simulink model "sm_i2c_expansion"  (Simulink 9.2)
settings: Solver=VariableStepAuto  StartTime=0.0  StopTime=10.0  RelTol=1e-3
undefined symbols (not defined in the file): slave_i2c
libraries: haley_test_bench_lib x10, etherlab_lib x1
settings Model: Creator=entwicklungs-pc  LastModifiedBy=entwicklungs-pc
settings DataIOCC: LimitDataPoints=off  SaveFormat=Dataset  SignalLoggingSaveFormat=Dataset
settings OptimizationCC: LifeSpan=auto
settings DebuggingCC: UnderspecifiedInitializationDetection=Simplified  MergeDetectMultiDrivingBlocksExec=error  FcnCallInpInsideContextMsg=error  StateNameClashWarn=none  SFUnexpectedBacktrackingDiag=error  SFNoUnconditionalDefaultTransitionDiag=error  SFExecutionAtInitializationDiag=warning
settings HardwareCC: ProdBitPerPointer=64  ProdBitPerSizeT=64  ProdBitPerPtrDiffT=64  ProdLargestAtomicFloat=Float  ProdIntDivRoundTo=Zero  ProdEndianess=LittleEndian  ProdWordSize=64  ProdHWDeviceType=Intel->x86-64 (Windows64)
settings ModelReferenceCC: PropagateSignalLabelsOutOfModel=on
settings SFSimCC: SimUseLocalCustomCode=on
settings RTWCC: RTWUseLocalCustomCode=on
settings CodeAppCC: StateflowObjectComments=off
settings GRTTargetCC: TargetLangStandard=C99 (ISO)  GeneratePreprocessorConditionals=Use local settings  CombineOutputUpdateFcns=on  GRTInterface=off
settings ConfigComp: CovMetricSettings=dwe  CovHtmlReporting=off  CovSaveCumulativeToWorkspaceVar=off  CovSaveSingleToWorkspaceVar=off  CovExternalEMLEnable=on

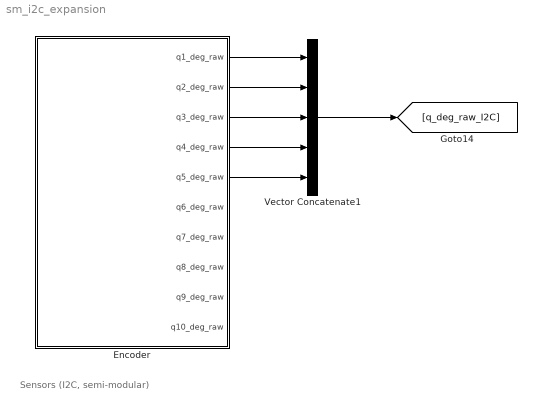
== system sm_i2c_expansion ==
  note: Sensors (I2C, semi-modular)
  Encoder : Subsystem
  Vector Concatenate1 : Concatenate  NumInputs=5
  wires:
  Encoder/1(q1_deg_raw) -> Vector Concatenate1/1
  Encoder/2(q2_deg_raw) -> Vector Concatenate1/2
  Encoder/5(q5_deg_raw) -> Vector Concatenate1/5
  Vector Concatenate1/1 -> [q_deg_raw_I2C]
  Encoder/3(q3_deg_raw) -> Vector Concatenate1/3
  Encoder/4(q4_deg_raw) -> Vector Concatenate1/4

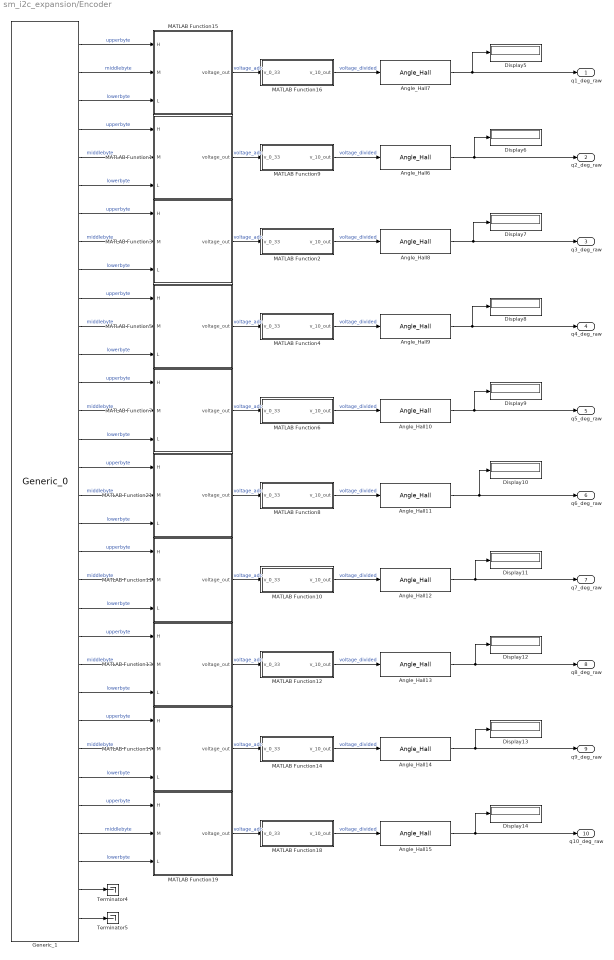
== system sm_i2c_expansion/Encoder ==
  Angle_Hall{6..15} (10 alike) : haley_test_bench_lib/Angle_Hall  SystemSampleTime=-1
  Display{5..14} (10 alike) : Display
  Generic_1 : etherlab_lib/EtherCAT/Generic_0  master=0  index=16  rv=slave_i2c()  param=[]  tsample=t_sample_s  debug=0
  MATLAB Function1 : MATLAB Function  TreatAsAtomicUnit=on
  MATLAB Function10 : MATLAB Function  TreatAsAtomicUnit=on
  MATLAB Function11 : MATLAB Function  TreatAsAtomicUnit=on
  MATLAB Function12 : MATLAB Function  TreatAsAtomicUnit=on
  MATLAB Function13 : MATLAB Function  TreatAsAtomicUnit=on
  MATLAB Function14 : MATLAB Function  TreatAsAtomicUnit=on
  MATLAB Function15 : MATLAB Function  TreatAsAtomicUnit=on
  MATLAB Function16 : MATLAB Function  TreatAsAtomicUnit=on
  MATLAB Function17 : MATLAB Function  TreatAsAtomicUnit=on
  MATLAB Function18 : MATLAB Function  TreatAsAtomicUnit=on
  MATLAB Function19 : MATLAB Function  TreatAsAtomicUnit=on
  MATLAB Function2 : MATLAB Function  TreatAsAtomicUnit=on
  MATLAB Function21 : MATLAB Function  TreatAsAtomicUnit=on
  MATLAB Function3 : MATLAB Function  TreatAsAtomicUnit=on
  MATLAB Function4 : MATLAB Function  TreatAsAtomicUnit=on
  MATLAB Function5 : MATLAB Function  TreatAsAtomicUnit=on
  MATLAB Function6 : MATLAB Function  TreatAsAtomicUnit=on
  MATLAB Function7 : MATLAB Function  TreatAsAtomicUnit=on
  MATLAB Function8 : MATLAB Function  TreatAsAtomicUnit=on
  MATLAB Function9 : MATLAB Function  TreatAsAtomicUnit=on
  Terminator4 : Terminator
  Terminator5 : Terminator
  q1_deg_raw : Outport
  q2_deg_raw : Outport  Port=2
  q3_deg_raw : Outport  Port=3
  q4_deg_raw : Outport  Port=4
  q5_deg_raw : Outport  Port=5
  q6_deg_raw : Outport  Port=6
  q7_deg_raw : Outport  Port=7
  q8_deg_raw : Outport  Port=8
  q9_deg_raw : Outport  Port=9
  q10_deg_raw : Outport  Port=10
  wires:
  MATLAB Function6/1(v_10_out) -> Angle_Hall10/1  "voltage_divided"
  Generic_1/3 -> MATLAB Function15/3(L)  "lowerbyte"
  Angle_Hall10/1 -> Display9/1, q5_deg_raw/1
  Angle_Hall6/1 -> q2_deg_raw/1, Display6/1
  MATLAB Function3/1(voltage_out) -> MATLAB Function2/1(v_0_33)  "voltage_adc"
  MATLAB Function2/1(v_10_out) -> Angle_Hall8/1  "voltage_divided"
  Generic_1/4 -> MATLAB Function1/1(H)  "upperbyte"
  Angle_Hall8/1 -> q3_deg_raw/1, Display7/1
  Generic_1/6 -> MATLAB Function1/3(L)  "lowerbyte"
  Generic_1/1 -> MATLAB Function15/1(H)  "upperbyte"
  MATLAB Function15/1(voltage_out) -> MATLAB Function16/1(v_0_33)  "voltage_adc"
  Generic_1/2 -> MATLAB Function15/2(M)  "middlebyte"
  Angle_Hall7/1 -> q1_deg_raw/1, Display5/1
  Generic_1/9 -> MATLAB Function3/3(L)  "lowerbyte"
  MATLAB Function5/1(voltage_out) -> MATLAB Function4/1(v_0_33)  "voltage_adc"
  MATLAB Function7/1(voltage_out) -> MATLAB Function6/1(v_0_33)  "voltage_adc"
  Generic_1/8 -> MATLAB Function3/2(M)  "middlebyte"
  MATLAB Function4/1(v_10_out) -> Angle_Hall9/1  "voltage_divided"
  MATLAB Function16/1(v_10_out) -> Angle_Hall7/1  "voltage_divided"
  MATLAB Function1/1(voltage_out) -> MATLAB Function9/1(v_0_33)  "voltage_adc"
  Generic_1/7 -> MATLAB Function3/1(H)  "upperbyte"
  Generic_1/10 -> MATLAB Function5/1(H)  "upperbyte"
  Generic_1/12 -> MATLAB Function5/3(L)  "lowerbyte"
  Angle_Hall9/1 -> q4_deg_raw/1, Display8/1
  Generic_1/13 -> MATLAB Function7/1(H)  "upperbyte"
  Generic_1/15 -> MATLAB Function7/3(L)  "lowerbyte"
  MATLAB Function9/1(v_10_out) -> Angle_Hall6/1  "voltage_divided"
  Generic_1/11 -> MATLAB Function5/2(M)  "middlebyte"
  Generic_1/14 -> MATLAB Function7/2(M)  "middlebyte"
  Generic_1/5 -> MATLAB Function1/2(M)  "middlebyte"
  Generic_1/16 -> MATLAB Function21/1(H)  "upperbyte"
  Generic_1/28 -> MATLAB Function19/1(H)  "upperbyte"
  MATLAB Function11/1(voltage_out) -> MATLAB Function10/1(v_0_33)  "voltage_adc"
  Generic_1/27 -> MATLAB Function17/3(L)  "lowerbyte"
  Generic_1/22 -> MATLAB Function13/1(H)  "upperbyte"
  MATLAB Function13/1(voltage_out) -> MATLAB Function12/1(v_0_33)  "voltage_adc"
  Generic_1/23 -> MATLAB Function13/2(M)  "middlebyte"
  Generic_1/20 -> MATLAB Function11/2(M)  "middlebyte"
  Generic_1/18 -> MATLAB Function21/3(L)  "lowerbyte"
  MATLAB Function19/1(voltage_out) -> MATLAB Function18/1(v_0_33)  "voltage_adc"
  Generic_1/29 -> MATLAB Function19/2(M)  "middlebyte"
  Generic_1/26 -> MATLAB Function17/2(M)  "middlebyte"
  Generic_1/21 -> MATLAB Function11/3(L)  "lowerbyte"
  MATLAB Function17/1(voltage_out) -> MATLAB Function14/1(v_0_33)  "voltage_adc"
  Generic_1/19 -> MATLAB Function11/1(H)  "upperbyte"
  MATLAB Function14/1(v_10_out) -> Angle_Hall14/1  "voltage_divided"
  Angle_Hall11/1 -> q6_deg_raw/1, Display10/1
  MATLAB Function21/1(voltage_out) -> MATLAB Function8/1(v_0_33)  "voltage_adc"
  Angle_Hall15/1 -> q10_deg_raw/1, Display14/1
  Generic_1/24 -> MATLAB Function13/3(L)  "lowerbyte"
  MATLAB Function18/1(v_10_out) -> Angle_Hall15/1  "voltage_divided"
  Generic_1/30 -> MATLAB Function19/3(L)  "lowerbyte"
  Generic_1/17 -> MATLAB Function21/2(M)  "middlebyte"
  MATLAB Function12/1(v_10_out) -> Angle_Hall13/1  "voltage_divided"
  Generic_1/25 -> MATLAB Function17/1(H)  "upperbyte"
  Angle_Hall12/1 -> q7_deg_raw/1, Display11/1
  MATLAB Function8/1(v_10_out) -> Angle_Hall11/1  "voltage_divided"
  Angle_Hall13/1 -> q8_deg_raw/1, Display12/1
  Angle_Hall14/1 -> q9_deg_raw/1, Display13/1
  MATLAB Function10/1(v_10_out) -> Angle_Hall12/1  "voltage_divided"
  Generic_1/32 -> Terminator5/1
  Generic_1/31 -> Terminator4/1

== matlab function Encoder/MATLAB Function1 ==
  data: H input uint8 size=1; M input double; L input uint8 size=1; voltage_out output double size=1
function voltage_out = concat_bitwise(H, M, L)

    raw_value = double(bitshift(int32(H), 16) + bitshift(int32(M), 8) + int32(L));  

    % Convert raw ADC value to voltage
    voltage_out = (3.333333333333333333 / 8388607) * raw_value; 
end

== matlab function Encoder/MATLAB Function2 ==
  data: v_0_33 input double; v_10_out output double
function v_10_out = map_voltage(v_0_33)
%reconstruct output voltage after voltage divider
v_10_out = v_0_33*(1+2)/1; %divider: V_0_33 = V_10*R_2/(R_1+R_2) --- R1 = 200kOhm, R2=100kOhm

== matlab function Encoder/MATLAB Function3 ==
  data: H input uint8 size=1; M input double; L input uint8 size=1; voltage_out output double size=1
function voltage_out = concat_bitwise(H, M, L)

    raw_value = double(bitshift(int32(H), 16) + bitshift(int32(M), 8) + int32(L));  

    % Convert raw ADC value to voltage
    voltage_out = (3.333333333333333333 / 8388607) * raw_value; 
end

== matlab function Encoder/MATLAB Function4 ==
  data: v_0_33 input double; v_10_out output double
function v_10_out = map_voltage(v_0_33)
%reconstruct output voltage after voltage divider
v_10_out = v_0_33*(1+2)/1; %divider: V_0_33 = V_10*R_2/(R_1+R_2) --- R1 = 200kOhm, R2=100kOhm

== matlab function Encoder/MATLAB Function5 ==
  data: H input uint8 size=1; M input double; L input uint8 size=1; voltage_out output double size=1
function voltage_out = concat_bitwise(H, M, L)

    raw_value = double(bitshift(int32(H), 16) + bitshift(int32(M), 8) + int32(L));  

    % Convert raw ADC value to voltage
    voltage_out = (3.333333333333333333 / 8388607) * raw_value; 
end

== matlab function Encoder/MATLAB Function6 ==
  data: v_0_33 input double; v_10_out output double
function v_10_out = map_voltage(v_0_33)
%reconstruct output voltage after voltage divider
v_10_out = v_0_33*(1+2)/1; %divider: V_0_33 = V_10*R_2/(R_1+R_2) --- R1 = 200kOhm, R2=100kOhm

== matlab function Encoder/MATLAB Function7 ==
  data: H input uint8 size=1; M input double; L input uint8 size=1; voltage_out output double size=1
function voltage_out = concat_bitwise(H, M, L)

    raw_value = double(bitshift(int32(H), 16) + bitshift(int32(M), 8) + int32(L));  

    % Convert raw ADC value to voltage
    voltage_out = (3.333333333333333333 / 8388607) * raw_value; 
end

== matlab function Encoder/MATLAB Function8 ==
  data: v_0_33 input double; v_10_out output double
function v_10_out = map_voltage(v_0_33)
%reconstruct output voltage after voltage divider
v_10_out = v_0_33*(1+2)/1; %divider: V_0_33 = V_10*R_2/(R_1+R_2) --- R1 = 200kOhm, R2=100kOhm

== matlab function Encoder/MATLAB Function9 ==
  data: v_0_33 input double; v_10_out output double
function v_10_out = map_voltage(v_0_33)
%reconstruct output voltage after voltage divider
v_10_out = v_0_33*(1+2)/1; %divider: V_0_33 = V_10*R_2/(R_1+R_2) --- R1 = 200kOhm, R2=100kOhm

== matlab function Encoder/MATLAB Function10 ==
  data: v_0_33 input double; v_10_out output double
function v_10_out = map_voltage(v_0_33)
%reconstruct output voltage after voltage divider
v_10_out = v_0_33*(1+2)/1; %divider: V_0_33 = V_10*R_2/(R_1+R_2) --- R1 = 200kOhm, R2=100kOhm

== matlab function Encoder/MATLAB Function11 ==
  data: H input uint8 size=1; M input double; L input uint8 size=1; voltage_out output double size=1
function voltage_out = concat_bitwise(H, M, L)

    raw_value = double(bitshift(int32(H), 16) + bitshift(int32(M), 8) + int32(L));  

    % Convert raw ADC value to voltage
    voltage_out = (3.333333333333333333 / 8388607) * raw_value; 
end

== matlab function Encoder/MATLAB Function21 ==
  data: H input uint8 size=1; M input double; L input uint8 size=1; voltage_out output double size=1
function voltage_out = concat_bitwise(H, M, L)

    raw_value = double(bitshift(int32(H), 16) + bitshift(int32(M), 8) + int32(L));  

    % Convert raw ADC value to voltage
    voltage_out = (3.333333333333333333 / 8388607) * raw_value; 
end

== matlab function Encoder/MATLAB Function12 ==
  data: v_0_33 input double; v_10_out output double
function v_10_out = map_voltage(v_0_33)
%reconstruct output voltage after voltage divider
v_10_out = v_0_33*(1+2)/1; %divider: V_0_33 = V_10*R_2/(R_1+R_2) --- R1 = 200kOhm, R2=100kOhm

== matlab function Encoder/MATLAB Function13 ==
  data: H input uint8 size=1; M input double; L input uint8 size=1; voltage_out output double size=1
function voltage_out = concat_bitwise(H, M, L)

    raw_value = double(bitshift(int32(H), 16) + bitshift(int32(M), 8) + int32(L));  

    % Convert raw ADC value to voltage
    voltage_out = (3.333333333333333333 / 8388607) * raw_value; 
end

== matlab function Encoder/MATLAB Function14 ==
  data: v_0_33 input double; v_10_out output double
function v_10_out = map_voltage(v_0_33)
%reconstruct output voltage after voltage divider
v_10_out = v_0_33*(1+2)/1; %divider: V_0_33 = V_10*R_2/(R_1+R_2) --- R1 = 200kOhm, R2=100kOhm

== matlab function Encoder/MATLAB Function17 ==
  data: H input uint8 size=1; M input double; L input uint8 size=1; voltage_out output double size=1
function voltage_out = concat_bitwise(H, M, L)

    raw_value = double(bitshift(int32(H), 16) + bitshift(int32(M), 8) + int32(L));  

    % Convert raw ADC value to voltage
    voltage_out = (3.333333333333333333 / 8388607) * raw_value; 
end

== matlab function Encoder/MATLAB Function18 ==
  data: v_0_33 input double; v_10_out output double
function v_10_out = map_voltage(v_0_33)
%reconstruct output voltage after voltage divider
v_10_out = v_0_33*(1+2)/1; %divider: V_0_33 = V_10*R_2/(R_1+R_2) --- R1 = 200kOhm, R2=100kOhm

== matlab function Encoder/MATLAB Function19 ==
  data: H input uint8 size=1; M input double; L input uint8 size=1; voltage_out output double size=1
function voltage_out = concat_bitwise(H, M, L)

    raw_value = double(bitshift(int32(H), 16) + bitshift(int32(M), 8) + int32(L));  

    % Convert raw ADC value to voltage
    voltage_out = (3.333333333333333333 / 8388607) * raw_value; 
end

== matlab function Encoder/MATLAB Function15 ==
  data: H input uint8 size=1; M input double; L input uint8 size=1; voltage_out output double size=1
function voltage_out = concat_bitwise(H, M, L)

    raw_value = double(bitshift(int32(H), 16) + bitshift(int32(M), 8) + int32(L));  

    % Convert raw ADC value to voltage
    voltage_out = (3.333333333333333333 / 8388607) * raw_value; 
end

== matlab function Encoder/MATLAB Function16 ==
  data: v_0_33 input double; v_10_out output double
function v_10_out = map_voltage(v_0_33)
%reconstruct output voltage after voltage divider
v_10_out = v_0_33*(1+2)/1; %divider: V_0_33 = V_10*R_2/(R_1+R_2) --- R1 = 200kOhm, R2=100kOhm
